simulink model "dym_val"  (R2024b)
settings: Solver=VariableStepAuto  StartTime=0.0  StopTime=200  RelTol=1e-3
libraries: dspinverses x1, Mako_Dynamics x1
settings Model: Creator=pinto  LastModifiedBy=pinto

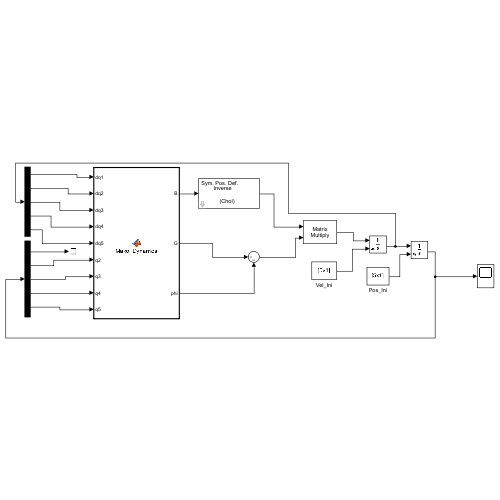
[thumbnail: Simulink's stored preview of the top-level diagram]
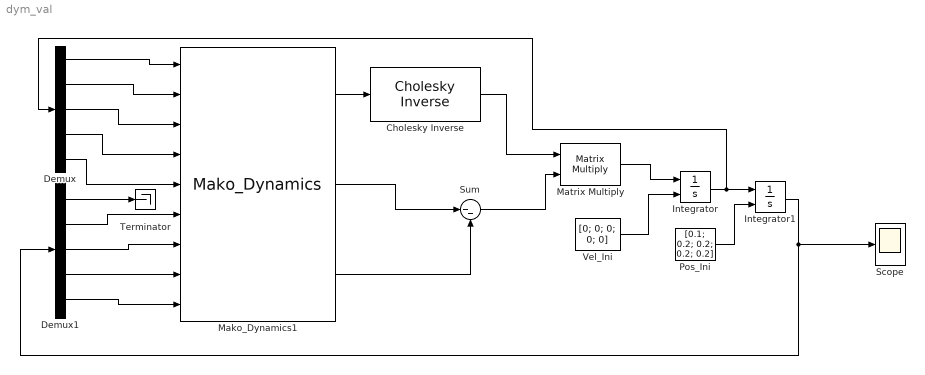
== system dym_val ==
  Cholesky Inverse : dspinverses/Cholesky Inverse  errmode=Warning
  Demux : Demux  Outputs=5
  Demux1 : Demux  Outputs=5
  Integrator : Integrator  InitialConditionSource=external  InitialCondition=[0.01, 0.01, 0.01]
  Integrator1 : Integrator  InitialConditionSource=external  InitialCondition=[0.01, 0.01, 0.01]
  Mako_Dynamics1 : Mako_Dynamics/Mako_Dynamics  SystemSampleTime=-1  VariantActivationTime=update diagram  AllowFlexibleInterface=on  Latency=0  AutoFrameSizeCalculation=off
  Matrix Multiply : Product  Multiplication=Matrix(*)
  Pos_Ini : Constant  Value=[0.1; 0.2; 0.2; 0.2; 0.2]
  Scope : Scope
  Sum : Sum  Inputs=|--
  Terminator : Terminator
  Vel_Ini : Constant  Value=[0; 0; 0; 0; 0]
  wires:
  Sum/1 -> Matrix Multiply/2
  Integrator1/1 -> Demux1/1, Scope/1
  Demux1/4 -> Mako_Dynamics1/8
  Mako_Dynamics1/1 -> Cholesky Inverse/1
  Demux/5 -> Mako_Dynamics1/5
  Demux1/2 -> Mako_Dynamics1/6
  Demux1/1 -> Terminator/1
  Cholesky Inverse/1 -> Matrix Multiply/1
  Mako_Dynamics1/2 -> Sum/1
  Demux1/5 -> Mako_Dynamics1/9
  Matrix Multiply/1 -> Integrator/1
  Demux1/3 -> Mako_Dynamics1/7
  Demux/1 -> Mako_Dynamics1/1
  Vel_Ini/1 -> Integrator/2
  Demux/4 -> Mako_Dynamics1/4
  Demux/3 -> Mako_Dynamics1/3
  Integrator/1 -> Integrator1/1, Demux/1
  Demux/2 -> Mako_Dynamics1/2
  Mako_Dynamics1/3 -> Sum/2
  Pos_Ini/1 -> Integrator1/2
